simulink model "PECT08"  (R2015b)
settings: Solver=FixedStepAuto  StartTime=0.0  StopTime=100  RelTol=1e-3
undefined symbols (not defined in the file): PDRref, sigbuilder_block
libraries: slrtlib x13, xpcnilib x11, simulink x9, dspfdesign x7, simulink_extras x1
(part 3 of 3)

== matlab function PECT08/oilrig setup1/terminating_safety/err_low ==
  data: chk input; sensnames input uint8; stop output
function stop  = fcn(chk, sensnames)
%#codegen
test = char(sensnames.');
k = strfind(test, '/');
k = [0 k];
k = [k numel(sensnames)];
stop = 0;
for i = 1:numel(chk)
    if chk(i) == 0
        str = char(test(k(i)+1:k(i+1)-1));
        Error = [str ': VALUE TOO LOW']
        coder.ceval('printf', ['%s' 10 0], Error);
        stop = stop+1;
    end
end
